simulink model "lab09"  (R2014a)
settings: Solver=ode45  StartTime=0.0  StopTime=40  RelTol=1e-3
libraries: commrandsrc2 x1, dspsrcs4 x1
settings Model: Creator=郑祖闯  LastModifiedBy=郑祖闯

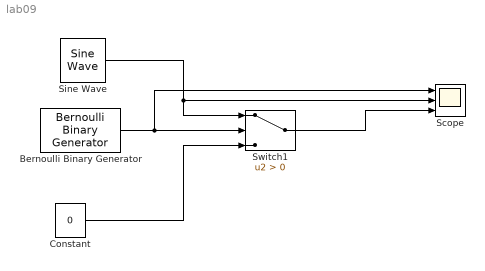
== system lab09 ==
  Bernoulli Binary Generator : commrandsrc2/Bernoulli Binary Generator  P=0.5  seed=61  Ts=1  frameBased=off  sampPerFrame=1  orient=off  outDataType=double
  Constant : Constant  Value=0  VectorParams1D=off
  Scope : Scope  NumInputPorts=3
      settings: TickLabels=on  TimeRange=40  YMin=-2~-2~-2  YMax=2~2~2
  Sine Wave : dspsrcs4/Sine Wave  Amplitude=1  Frequency=2  Phase=0  SampleMode=Discrete  OutComplex=Real  CompMethod=Trigonometric fcn  TableSize=Speed  SampleTime=1/50  SamplesPerFrame=1  ResetState=Restart at time zero  dataType=double  wordLen=16  udDataType=sfix(16)  fracBitsMode=Best precision  numFracBits=15  OutDataTypeStr=double  LastOutDataTypeStr=double
  Switch1 : Switch  Criteria=u2 > Threshold
  wires:
  Bernoulli Binary Generator/1 -> Scope/1, Switch1/2
  Sine Wave/1 -> Scope/2, Switch1/1
  Constant/1 -> Switch1/3
  Switch1/1 -> Scope/3
